simulink model "closed_loop2"  (R2021b)
settings: Solver=ode4  StartTime=0.0  StopTime=64  FixedStep=0.005  RelTol=1e-3
values from neighbouring files (symbols this model uses):
  A = [0        0                     1               0 ... (first row only)    [IP.m]    (also in IP_experiment.m; IP_sim.m)
  B = [         0 ... (first row only)    [IP.m]    (also in IP_experiment.m; IP_sim.m)
  C = eye(4)    [IP.m]    (also in IP_experiment.m = [1 0 0 0; IP_sim.m = [1 0 0 0)
  D = zeros(4, 1)    [IP.m]    (also in IP_experiment.m = [0;0]; IP_sim.m = [0;0])
  LPF_A = [0              1           0               0 ... (first row only)    [IP_experiment.m]    (also in IP_sim.m)
  LPF_B = [                    0                           0 ... (first row only)    [IP_experiment.m]    (also in IP_sim.m)
  LPF_C = [-1/T_s    1/T_s         0         0 ... (first row only)    [IP_experiment.m]    (also in IP_sim.m)
  LPF_D = zeros(2)    [IP_experiment.m]    (also in IP_sim.m)
  rnd = randi(500, 1)    [IP_experiment.m]    (also in IP_sim.m)
  x0 = [pos_init  angle_init  0   0]'    [IP.m]    (also in IP_experiment.m = [pos_init  angle_init      0.0     0.0]; IP_sim.m = [pos_init  angle_init      0.0     0.0])
undefined symbols (not defined in the file or in its folder): K
libraries: simulink x2
settings Model: Creator=yz  LastModifiedBy=yz

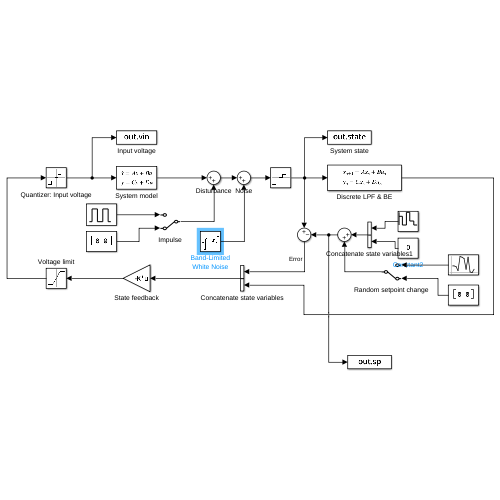
[thumbnail: Simulink's stored preview of the top-level diagram]
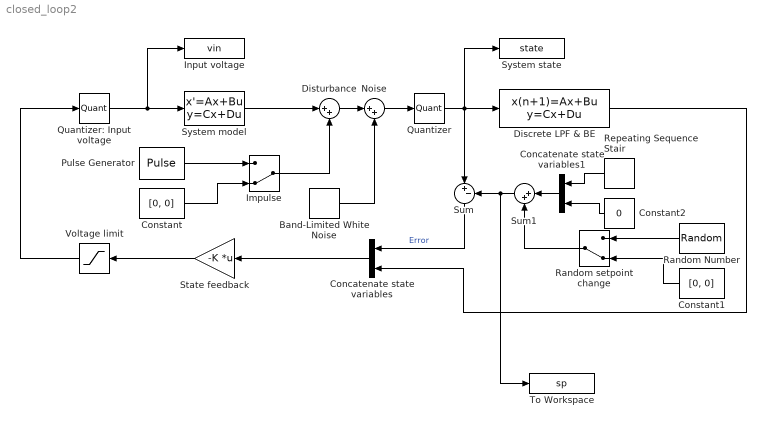
== system closed_loop2 ==
  Band-Limited White Noise : simulink/Sources/Band-Limited White Noise  Cov=[1e-8, 1e-8]  Ts=0.01  seed=[23341]
  Concatenate state variables : Concatenate
  Concatenate state variables1 : Concatenate
  Constant : Constant  Value=[0, 0]
  Constant1 : Constant  Value=[0, 0]
  Constant2 : Constant  Value=0  SampleTime=0.005
  Discrete LPF & BE : DiscreteStateSpace  A=LPF_A  B=LPF_B  C=LPF_C  D=LPF_D  InitialCondition=[0,0,0,0]  SampleTime=-1
  Disturbance : Sum  Inputs=|++
  Impulse : ManualSwitch  CurrentSetting=0
  Input voltage : ToWorkspace  VariableName=vin  SampleTime=-1
  Noise : Sum  Inputs=|++
  Pulse Generator : DiscretePulseGenerator  PulseType=Time based  Amplitude=[0, 0.5]  Period=5  PulseWidth=0.2  PhaseDelay=2
  Quantizer : Quantizer  QuantizationInterval=20/65536
  Quantizer: Input voltage : Quantizer  QuantizationInterval=10/65536
  Random Number : RandomNumber  Mean=[0, 0]  Variance=[0.04, 0]  Seed=rnd  SampleTime=8
  Random setpoint change : ManualSwitch  CurrentSetting=0
  Repeating Sequence Stair : simulink/Sources/Repeating Sequence Stair  OutValues=xd  tsamp=0.005  OutMin=[]  OutMax=[]  OutDataTypeStr=double  OutputDataTypeScalingMode=double  OutDataType=fixdt(0,8)  ConRadixGroup=Best Precision: Vector-wise  OutScaling=2^-12
  State feedback : Gain  Gain=-K  Multiplication=Matrix(K*u)
  Sum : Sum  Inputs=|+-
  Sum1 : Sum  Inputs=|++
  System model : StateSpace  A=A  B=B  C=C  D=D  InitialCondition=x0
  System state : ToWorkspace  VariableName=state  SampleTime=-1
  To Workspace : ToWorkspace  VariableName=sp  SampleTime=0.005
  Voltage limit : Saturate  UpperLimit=5  LowerLimit=-5
  wires:
  System model/1 -> Disturbance/1
  Impulse/1 -> Disturbance/2
  Constant/1 -> Impulse/2
  State feedback/1 -> Voltage limit/1
  Voltage limit/1 -> Quantizer: Input voltage/1
  Sum/1 -> Concatenate state variables/1  "Error"
  Concatenate state variables/1 -> State feedback/1
  Discrete LPF & BE/1 -> Concatenate state variables/2
  Quantizer/1 -> System state/1, Discrete LPF & BE/1, Sum/1
  Quantizer: Input voltage/1 -> System model/1, Input voltage/1
  Pulse Generator/1 -> Impulse/1
  Sum1/1 -> Sum/2, To Workspace/1
  Random Number/1 -> Random setpoint change/1
  Random setpoint change/1 -> Sum1/2
  Constant1/1 -> Random setpoint change/2
  Disturbance/1 -> Noise/1
  Noise/1 -> Quantizer/1
  Band-Limited White Noise/1 -> Noise/2
  Concatenate state variables1/1 -> Sum1/1
  Repeating Sequence Stair/1 -> Concatenate state variables1/1
  Constant2/1 -> Concatenate state variables1/2
